simulink library "command_processing"  (R2016b)
settings: Solver=VariableStepAuto  StartTime=0.0  StopTime=10.0  RelTol=1e-3
undefined symbols (not defined in the file or in its folder): fsw_params
settings Model: Creator=taylorreynolds  LastModifiedBy=Taylor

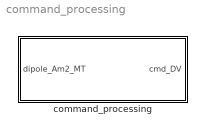
== system command_processing ==
  command_processing : Subsystem

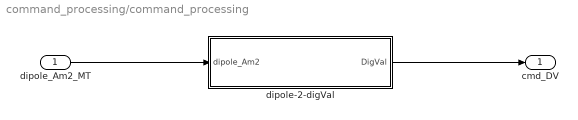
== system command_processing/command_processing ==
  dipole_Am2_MT : Inport
  dipole-2-digVal : Subsystem
  cmd_DV : Outport
  wires:
  dipole_Am2_MT/1 -> dipole-2-digVal/1(dipole_Am2)
  dipole-2-digVal/1(DigVal) -> cmd_DV/1

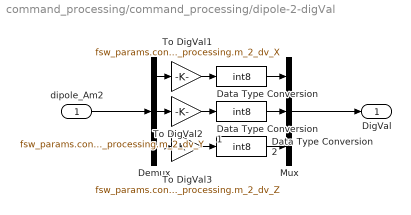
== system command_processing/command_processing/dipole-2-digVal ==
  dipole_Am2 : Inport
  Data Type Conversion : DataTypeConversion  OutDataTypeStr=int8  RndMeth=Nearest
  Data Type Conversion1 : DataTypeConversion  OutDataTypeStr=int8  RndMeth=Nearest
  Data Type Conversion2 : DataTypeConversion  OutDataTypeStr=int8  RndMeth=Nearest
  Demux : Demux  Outputs=3
  Mux : Mux  Inputs=3
  To DigVal1 : Gain  Gain=fsw_params.control.cmd_processing.m_2_dv_X
  To DigVal2 : Gain  Gain=fsw_params.control.cmd_processing.m_2_dv_Y
  To DigVal3 : Gain  Gain=fsw_params.control.cmd_processing.m_2_dv_Z
  DigVal : Outport
  wires:
  dipole_Am2/1 -> Demux/1
  Demux/3 -> To DigVal3/1
  Demux/2 -> To DigVal2/1
  Demux/1 -> To DigVal1/1
  To DigVal1/1 -> Data Type Conversion/1
  To DigVal2/1 -> Data Type Conversion1/1
  To DigVal3/1 -> Data Type Conversion2/1
  Mux/1 -> DigVal/1
  Data Type Conversion/1 -> Mux/1
  Data Type Conversion1/1 -> Mux/2
  Data Type Conversion2/1 -> Mux/3
